simulink model "model"  (R2020b)
settings: Solver=VariableStepAuto  StartTime=0.0  StopTime=10.0  RelTol=1e-3
model workspace (MAT data in the model file):
  Ts = Simulink.Parameter
  Ts.Value = 0.01
  Ts.DataType = 'auto'
  Ts.Dimensions = [1 1]
values from neighbouring files (symbols this model uses):
  b = 50.0    [motor_speed_data.sldd]
  m = 1000.0    [motor_speed_data.sldd]
settings Model: Creator=Lenovo  LastModifiedBy=Lenovo

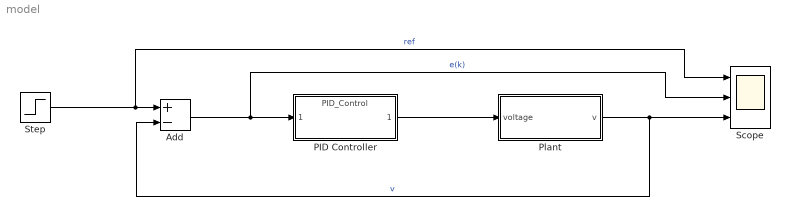
== system model ==
  Add : Sum  Inputs=+-
  PID Controller : ModelReference  ModelNameDialog=PID_Control  UsingDefaultArgumentValue=0,0,0  SimulationMode=Normal  ModelReferenceVersion=1.6  Kp=0  Ki=0  Kd=0  SimulationMode=Normal
  Plant : Subsystem
  Scope : Scope  NumInputPorts=3
  Step : Step  SampleTime=0
  wires:
  Plant/1(v) -> Add/2, Scope/3  "v"
  PID Controller/1 -> Plant/1(voltage)
  Add/1 -> PID Controller/1, Scope/2  "e(k)"
  Step/1 -> Add/1, Scope/1  "ref"

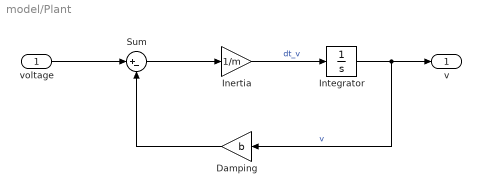
== system model/Plant ==
  voltage : Inport
  Damping : Gain  Gain=b
  Inertia : Gain  Gain=1/m
  Integrator : Integrator
  Sum : Sum  Inputs=|+-
  v : Outport
  wires:
  Damping/1 -> Sum/2
  voltage/1 -> Sum/1
  Sum/1 -> Inertia/1
  Inertia/1 -> Integrator/1  "dt_v"
  Integrator/1 -> Damping/1, v/1  "v"
